simulink model "simulinkFluj"  (R2023b)
settings: Solver=ode4  StartTime=0.0  StopTime=50  FixedStep=1e-3  RelTol=1e-3
libraries: cstblocks x3
settings Model: Creator=daas0  LastModifiedBy=daas0

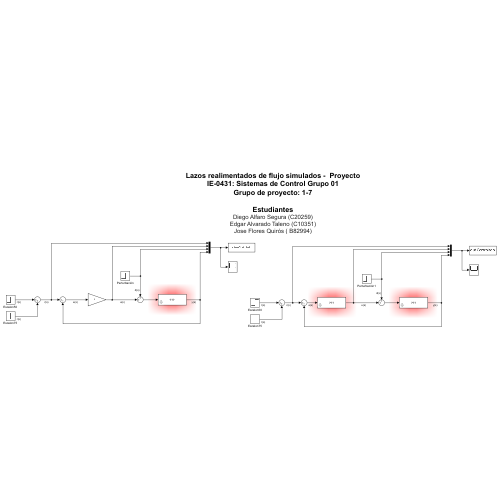
[thumbnail: Simulink's stored preview of the top-level diagram]
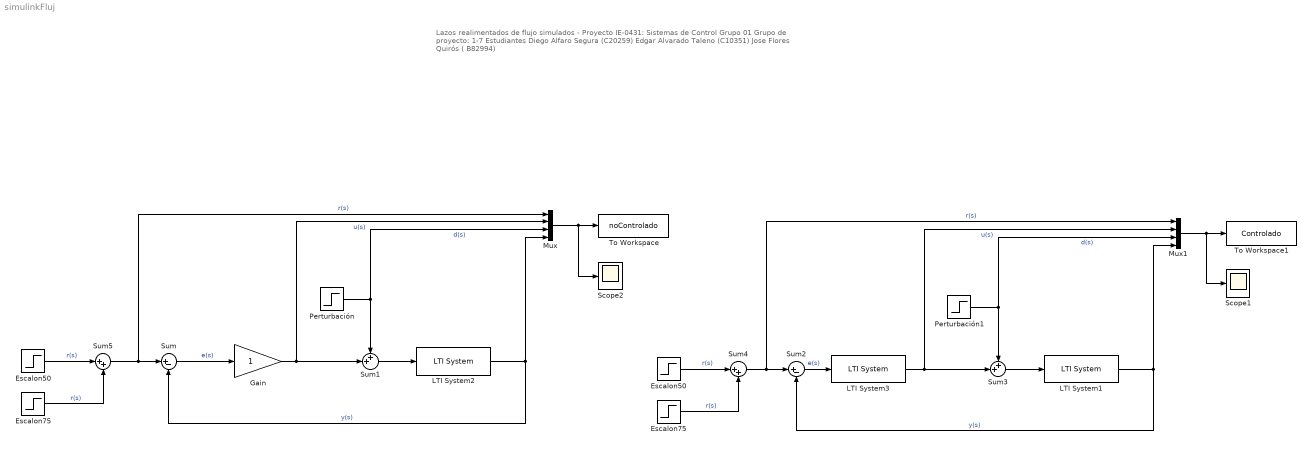
== system simulinkFluj ==
  note: Lazos realimentados de flujo simulados - Proyecto
      | IE-0431: Sistemas de Control Grupo 01
      | Grupo de proyecto: 1-7
      |
      | Estudiantes
      | Diego Alfaro Segura (C20259)
      | Edgar Alvarado Taleno (C10351)
      | Jose Flores Quirós ( B82994)
  Escalon50 : Step  Time=0  After=50  SampleTime=0
  "Escalon50 " : Step  Time=0  After=50  SampleTime=0
  Escalon75 : Step  Time=20  After=25  SampleTime=0
  "Escalon75 " : Step  Time=20  After=25  SampleTime=0
  Gain : Gain
  LTI System1 : cstblocks/LTI System  sys=fluj_G  IC=[]  PadeOrder=0
  LTI System2 : cstblocks/LTI System  sys=fluj_G  IC=[]  PadeOrder=0
  LTI System3 : cstblocks/LTI System  sys=controladorPID  IC=[]  PadeOrder=0
  Mux : Mux
  Mux1 : Mux
  Perturbación : Step  Time=40  After=20  SampleTime=0
  Perturbación1 : Step  Time=40  After=20  SampleTime=0
  Scope1 : Scope
  Scope2 : Scope
  Sum : Sum  Inputs=|+-
  Sum1 : Sum  Inputs=++|
  Sum2 : Sum  Inputs=|+-
  Sum3 : Sum  Inputs=++|
  Sum4 : Sum  Inputs=|++
  Sum5 : Sum  Inputs=|++
  To Workspace : ToWorkspace  VariableName=noControlado  SaveFormat=Timeseries  SampleTime=-1
  To Workspace1 : ToWorkspace  VariableName=Controlado  SaveFormat=Timeseries  SampleTime=-1
  wires:
  LTI System2/1 -> Mux/4, Sum/2  "y(s)"
  Sum/1 -> Gain/1  "e(s)"
  Sum5/1 -> Mux/1, Sum/1  "r(s)"
  Gain/1 -> Mux/2, Sum1/2  "u(s)"
  Sum1/1 -> LTI System2/1
  Perturbación/1 -> Sum1/1, Mux/3  "d(s)"
  Mux/1 -> Scope2/1, To Workspace/1
  Mux1/1 -> Scope1/1, To Workspace1/1
  Perturbación1/1 -> Sum3/1, Mux1/3  "d(s)"
  Sum4/1 -> Mux1/1, Sum2/1  "r(s)"
  LTI System1/1 -> Mux1/4, Sum2/2  "y(s)"
  Sum2/1 -> LTI System3/1  "e(s)"
  LTI System3/1 -> Mux1/2, Sum3/2  "u(s)"
  Sum3/1 -> LTI System1/1
  Escalon75/1 -> Sum4/2  "r(s)"
  Escalon50/1 -> Sum4/1  "r(s)"
  "Escalon75 "/1 -> Sum5/2  "r(s)"
  "Escalon50 "/1 -> Sum5/1  "r(s)"
